simulink model "p_regulator"  (R2019b)
settings: Solver=VariableStepAuto  StartTime=0.0  StopTime=10.0  RelTol=1e-3
undefined symbols (not defined in the file): J, km, L, R
settings Model: Creator=Gudini  LastModifiedBy=Gudini

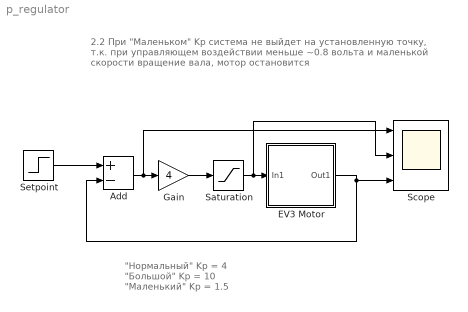
== system p_regulator ==
  note: 2.2
      | При "Маленьком" Kp система не выйдет на установленную точку,
      |  т.к. при управляющем воздействии меньше ~0.8 вольта
      |  и маленькой скорости вращение вала, мотор остановится
  note: "Нормальный" Kp = 4
      | "Большой" Kp = 10
      | "Маленький" Kp = 1.5
  Add : Sum  Inputs=+-
  EV3 Motor : Subsystem
  Gain : Gain  Gain=4
  Saturation : Saturate  UpperLimit=7.6  LowerLimit=-7.6
  Scope : Scope  NumInputPorts=3
  "Setpoint " : Step  After=3.14  SampleTime=0
  wires:
  EV3 Motor/1(Out1) -> Add/2, Scope/3
  Add/1 -> Scope/1, Gain/1
  Gain/1 -> Saturation/1
  "Setpoint "/1 -> Add/1
  Saturation/1 -> Scope/2, EV3 Motor/1(In1)

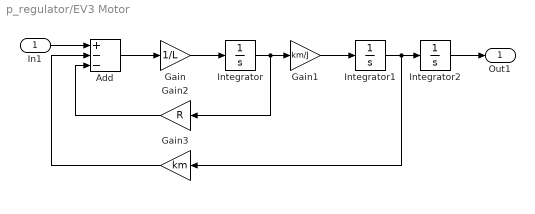
== system p_regulator/EV3 Motor ==
  In1 : Inport
  Add : Sum  Inputs=+--
  Gain : Gain  Gain=1/L
  Gain1 : Gain  Gain=km/J
  Gain2 : Gain  Gain=R
  Gain3 : Gain  Gain=km
  Integrator : Integrator
  Integrator1 : Integrator
  Integrator2 : Integrator
  Out1 : Outport
  wires:
  Gain1/1 -> Integrator1/1
  Integrator1/1 -> Gain3/1, Integrator2/1
  In1/1 -> Add/1
  Integrator2/1 -> Out1/1
  Integrator/1 -> Gain2/1, Gain1/1
  Gain/1 -> Integrator/1
  Gain2/1 -> Add/3
  Add/1 -> Gain/1
  Gain3/1 -> Add/2
